simulink model "MotorDynamic"  (Simulink 7.4)
settings: Solver=ode45  StartTime=0.0  StopTime=60.0  MaxStep=0.002  RelTol=1e-3
values from neighbouring files (symbols this model uses):
  Bm = 0.00005299859    (= 5.299859e-05)    [A23150.m]    (also in Motor.mat; MotorDynamics.m = 8.920308e-05; MotorSimulationConfig.m; RS775Motor.m = 1.2515538461e-06)
  G_pwm = (1/128)    (= 0.0078125)    [MotorDynamics.m]
  kp = 1/300    (= 0.00333333333333)    [MotorDynamics.m]
  kt = 0.03552    [A23150.m]    (also in Motor.mat; MotorDynamics.m; RS775Motor.m = 0.009039)
  kv = KV1^(-1)    (= 0.0354992438529)    [A23150.m]    (also in Motor.mat; MotorDynamics.m = 0.03552; MotorSimulationConfig.m = 269; RS775Motor.m = 0.00881744838121)
  La = 0.068*10^(-3)    (= 6.8e-05)    [MotorDynamics.m]    (also in MotorSimulationConfig.m = 0.001)
  ra = 0.121    [MotorDynamics.m]    (also in MotorSimulationConfig.m = 0.21)
  tau_load = 0.0    (= 0)    [MotorDynamics.m]
undefined symbols (not defined in the file or in its folder): DiscIntNeverNeededParam
settings Model: Creator=Rabbitfox  LastModifiedBy=Rabbitfox

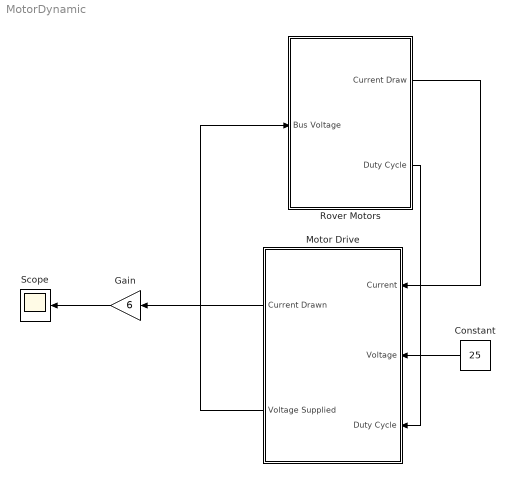
== system MotorDynamic ==
  Constant : Constant  Value=25  OutDataType=fixdt(1, 16)  OutScaling=2^0
  Gain : Gain  Gain=6  ParameterDataType=fixdt(1, 16)  ParameterScaling=2^0  OutDataType=fixdt(1, 16)  OutScaling=2^0
  Motor Drive : Subsystem
  Rover Motors : Subsystem
  Scope : Scope
      settings: SaveName=ScopeData2
  wires:
  Rover Motors/1(Current Draw) -> Motor Drive/1(Current)
  Motor Drive/2(Voltage Supplied) -> Rover Motors/1(Bus Voltage)
  Constant/1 -> Motor Drive/2(Voltage)
  Rover Motors/2(Duty Cycle) -> Motor Drive/3(Duty Cycle)
  Motor Drive/1(Current Drawn) -> Gain/1
  Gain/1 -> Scope/1

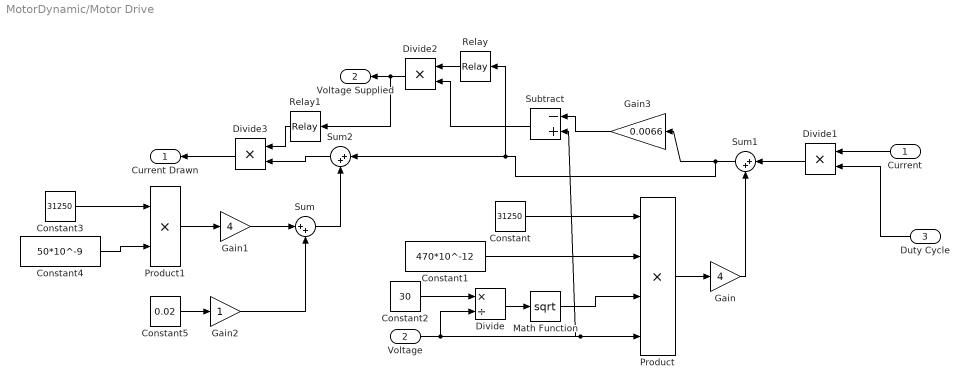
== system MotorDynamic/Motor Drive ==
  Current : Inport
  Voltage : Inport  Port=2
  Duty Cycle : Inport  Port=3
  Constant : Constant  Value=31250  OutDataType=fixdt(1, 16)  OutScaling=2^0
  Constant1 : Constant  Value=470*10^-12  OutDataType=fixdt(1, 16)  OutScaling=2^0
  Constant2 : Constant  Value=30  OutDataType=fixdt(1, 16)  OutScaling=2^0
  Constant3 : Constant  Value=31250  OutDataType=fixdt(1, 16)  OutScaling=2^0
  Constant4 : Constant  Value=50*10^-9  OutDataType=fixdt(1, 16)  OutScaling=2^0
  Constant5 : Constant  Value=0.02  OutDataType=fixdt(1, 16)  OutScaling=2^0
  Divide : Product  Inputs=*/  OutDataType=fixdt(1, 16)  OutScaling=2^-10
  Divide1 : Product  Inputs=**  OutDataType=fixdt(1, 16)  OutScaling=2^-10
  Divide2 : Product  Inputs=**  OutDataType=fixdt(1, 16)  OutScaling=2^-10
  Divide3 : Product  Inputs=**  OutDataType=fixdt(1, 16)  OutScaling=2^-10
  Gain : Gain  Gain=4  ParameterDataType=fixdt(1, 16)  ParameterScaling=2^0  OutDataType=fixdt(1, 16)  OutScaling=2^0
  Gain1 : Gain  Gain=4  ParameterDataType=fixdt(1, 16)  ParameterScaling=2^0  OutDataType=fixdt(1, 16)  OutScaling=2^0
  Gain2 : Gain  ParameterDataType=fixdt(1, 16)  ParameterScaling=2^0  OutDataType=fixdt(1, 16)  OutScaling=2^0
  Gain3 : Gain  Gain=0.0066  ParameterDataType=fixdt(1, 16)  ParameterScaling=2^0  OutDataType=fixdt(1, 16)  OutScaling=2^0
  Math Function : Math  Operator=sqrt  OutDataType=fixdt(1, 16)  OutScaling=2^0  SaturateOnIntegerOverflow=on
  Product : Product  Inputs=4  OutDataType=fixdt(1, 16)  OutScaling=2^0  RndMeth=Zero
  Product1 : Product  OutDataType=fixdt(1, 16)  OutScaling=2^0  RndMeth=Zero
  Relay : Relay  OnSwitchValue=12.5  OffSwitchValue=12.4  OnOutputValue=0  OffOutputValue=1  OutDataType=fixdt(1, 16)  OutScaling=2^0
  Relay1 : Relay  OnSwitchValue=1.5  OffSwitchValue=1  OutDataType=fixdt(1, 16)  OutScaling=2^0
  Subtract : Sum  Inputs=-+  OutDataType=fixdt(1, 16)  OutScaling=2^-10
  Sum : Sum  Inputs=|++  OutDataType=fixdt(1, 16)  OutScaling=2^0
  Sum1 : Sum  Inputs=|++  OutDataType=fixdt(1, 16)  OutScaling=2^0
  Sum2 : Sum  Inputs=|++  OutDataType=fixdt(1, 16)  OutScaling=2^0
  Current Drawn : Outport
  Voltage Supplied : Outport  Port=2
  wires:
  Constant2/1 -> Divide/1
  Divide/1 -> Math Function/1
  Math Function/1 -> Product/3
  Constant1/1 -> Product/2
  Constant/1 -> Product/1
  Constant3/1 -> Product1/1
  Product1/1 -> Gain1/1
  Constant4/1 -> Product1/2
  Product/1 -> Gain/1
  Constant5/1 -> Gain2/1
  Gain1/1 -> Sum/1
  Gain2/1 -> Sum/2
  Sum1/1 -> Gain3/1, Sum2/1, Relay/1
  Gain/1 -> Sum1/2
  Sum/1 -> Sum2/2
  Voltage/1 -> Divide/2, Product/4, Subtract/2
  Gain3/1 -> Subtract/1
  Divide1/1 -> Sum1/1
  Current/1 -> Divide1/1
  Duty Cycle/1 -> Divide1/2
  Relay/1 -> Divide2/1
  Divide2/1 -> Voltage Supplied/1, Relay1/1
  Subtract/1 -> Divide2/2
  Relay1/1 -> Divide3/1
  Sum2/1 -> Divide3/2
  Divide3/1 -> Current Drawn/1

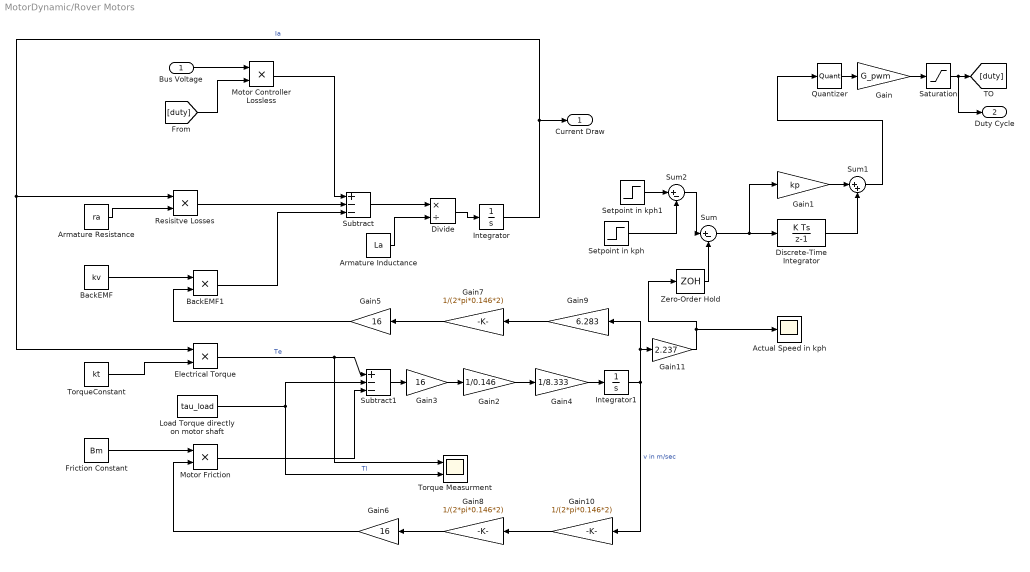
== system MotorDynamic/Rover Motors ==
  Bus Voltage : Inport  OutDataType=fixdt(1, 16)  OutScaling=2^0
  Actual Speed in kph : Scope
  Armature Inductance : Constant  Value=La  OutDataType=fixdt(1, 16)  OutScaling=2^0
  Armature Resistance : Constant  Value=ra  OutDataType=fixdt(1, 16)  OutScaling=2^0
  BackEMF : Constant  Value=kv  OutDataType=fixdt(1, 16)  OutScaling=2^0
  BackEMF1 : Product  OutDataType=fixdt(1, 16)  OutScaling=2^0  RndMeth=Zero
  Discrete-Time Integrator : DiscreteIntegrator  gainval=ki  SampleTime=sampletime  OutDataType=fixdt(1, 16)  OutScaling=2^0  LimitOutput=on  UpperSaturationLimit=128  LowerSaturationLimit=-128  ICPrevOutput=DiscIntNeverNeededParam  ICPrevScaledInput=DiscIntNeverNeededParam
  Divide : Product  Inputs=*/  OutDataType=fixdt(1, 16)  OutScaling=2^-10
  Electrical Torque : Product  OutDataType=fixdt(1, 16)  OutScaling=2^0  RndMeth=Zero
  Friction Constant : Constant  Value=Bm  OutDataType=fixdt(1, 16)  OutScaling=2^0
  Gain : Gain  Gain=G_pwm  ParameterDataType=fixdt(1, 16)  ParameterScaling=2^0  OutDataType=fixdt(1, 16)  OutScaling=2^0
  Gain1 : Gain  Gain=kp  ParameterDataType=fixdt(1, 16)  ParameterScaling=2^0  OutDataType=fixdt(1, 16)  OutScaling=2^0
  Gain10 : Gain  Gain=1/(2*pi*0.146*2)  ParameterDataType=fixdt(1, 16)  ParameterScaling=2^0  OutDataType=fixdt(1, 16)  OutScaling=2^0
  Gain11 : Gain  Gain=2.237  ParameterDataType=fixdt(1, 16)  ParameterScaling=2^0  OutDataType=fixdt(1, 16)  OutScaling=2^0
  Gain2 : Gain  Gain=1/0.146  ParameterDataType=fixdt(1, 16)  ParameterScaling=2^0  OutDataType=fixdt(1, 16)  OutScaling=2^0
  Gain3 : Gain  Gain=16  ParameterDataType=fixdt(1, 16)  ParameterScaling=2^0  OutDataType=fixdt(1, 16)  OutScaling=2^0
  Gain4 : Gain  Gain=1/8.333  ParameterDataType=fixdt(1, 16)  ParameterScaling=2^0  OutDataType=fixdt(1, 16)  OutScaling=2^0
  Gain5 : Gain  Gain=16  ParameterDataType=fixdt(1, 16)  ParameterScaling=2^0  OutDataType=fixdt(1, 16)  OutScaling=2^0
  Gain6 : Gain  Gain=16  ParameterDataType=fixdt(1, 16)  ParameterScaling=2^0  OutDataType=fixdt(1, 16)  OutScaling=2^0
  Gain7 : Gain  Gain=1/(2*pi*0.146*2)  ParameterDataType=fixdt(1, 16)  ParameterScaling=2^0  OutDataType=fixdt(1, 16)  OutScaling=2^0
  Gain8 : Gain  Gain=1/(2*pi*0.146*2)  ParameterDataType=fixdt(1, 16)  ParameterScaling=2^0  OutDataType=fixdt(1, 16)  OutScaling=2^0
  Gain9 : Gain  Gain=6.283  ParameterDataType=fixdt(1, 16)  ParameterScaling=2^0  OutDataType=fixdt(1, 16)  OutScaling=2^0
  Integrator : Integrator  UpperSaturationLimit=10  LowerSaturationLimit=-10
  Integrator1 : Integrator
  Load Torque directly on motor shaft : Constant  Value=tau_load  OutDataType=fixdt(1, 16)  OutScaling=2^0
  Motor Controller Lossless : Product  OutDataType=fixdt(1, 16)  OutScaling=2^0  RndMeth=Zero
  Motor Friction : Product  OutDataType=fixdt(1, 16)  OutScaling=2^0  RndMeth=Zero
  Quantizer : Quantizer  QuantizationInterval=1
  Resisitve Losses : Product  OutDataType=fixdt(1, 16)  OutScaling=2^0  RndMeth=Zero
  Saturation : Saturate  OutDataType=fixdt(1, 16)  OutScaling=2^0
  Setpoint in kph : Step  Time=30  After=.1  SampleTime=0
  Setpoint in kph1 : Step  Time=0.1  After=.1  SampleTime=0
  Subtract : Sum  Inputs=+--  OutDataType=fixdt(1, 16)  OutScaling=2^-10
  Subtract1 : Sum  Inputs=+--  OutDataType=fixdt(1, 16)  OutScaling=2^-10
  Sum : Sum  Inputs=|+-  OutDataType=fixdt(1, 16)  OutScaling=2^0
  Sum1 : Sum  Inputs=|++  OutDataType=fixdt(1, 16)  OutScaling=2^0
  Sum2 : Sum  Inputs=|+-  OutDataType=fixdt(1, 16)  OutScaling=2^0
  Torque Measurment : Scope  NumInputPorts=2
      settings: YMin=0.503~0.475  YMax=0.5095~0.525
  TorqueConstant : Constant  Value=kt  OutDataType=fixdt(1, 16)  OutScaling=2^0
  Zero-Order Hold : ZeroOrderHold  SampleTime=sampletime
  Current Draw : Outport  OutDataType=fixdt(1, 16)  OutScaling=2^0
  Duty Cycle : Outport  Port=2  OutDataType=fixdt(1, 16)  OutScaling=2^0
  wires:
  [duty] -> Motor Controller Lossless/2
  Friction Constant/1 -> Motor Friction/1
  Motor Friction/1 -> Subtract1/3
  Load Torque directly on motor shaft/1 -> Subtract1/2, Torque Measurment/2  "Tl"
  Electrical Torque/1 -> Torque Measurment/1, Subtract1/1  "Te"
  TorqueConstant/1 -> Electrical Torque/2
  Motor Controller Lossless/1 -> Subtract/1
  Bus Voltage/1 -> Motor Controller Lossless/1
  Integrator/1 -> Electrical Torque/1, Resisitve Losses/1, Current Draw/1  "Ia"
  Divide/1 -> Integrator/1
  Subtract/1 -> Divide/1
  BackEMF1/1 -> Subtract/3
  Resisitve Losses/1 -> Subtract/2
  Armature Inductance/1 -> Divide/2
  Armature Resistance/1 -> Resisitve Losses/2
  BackEMF/1 -> BackEMF1/1
  Quantizer/1 -> Gain/1
  Gain/1 -> Saturation/1
  Sum/1 -> Discrete-Time Integrator/1, Gain1/1
  Zero-Order Hold/1 -> Sum/2
  Saturation/1 -> [duty], Duty Cycle/1
  Discrete-Time Integrator/1 -> Sum1/2
  Gain1/1 -> Sum1/1
  Sum1/1 -> Quantizer/1
  Subtract1/1 -> Gain3/1
  Gain3/1 -> Gain2/1
  Gain2/1 -> Gain4/1
  Gain4/1 -> Integrator1/1
  Gain5/1 -> BackEMF1/2
  Gain6/1 -> Motor Friction/2
  Gain7/1 -> Gain5/1
  Gain8/1 -> Gain6/1
  Gain10/1 -> Gain8/1
  Gain9/1 -> Gain7/1
  Integrator1/1 -> Gain10/1, Gain9/1, Gain11/1  "v in m/sec"
  Gain11/1 -> Zero-Order Hold/1, Actual Speed in kph/1
  Setpoint in kph/1 -> Sum2/2
  Sum2/1 -> Sum/1
  Setpoint in kph1/1 -> Sum2/1
